simulink model "Filter_testaus_uusi"  (R2017b)
settings: Solver=FixedStepDiscrete  StartTime=0.0  StopTime=10  FixedStep=1/44100  RelTol=1e-3
(part 3 of 4)

== system Filter_testaus_uusi/Highpass/HighpassH/Resonator30 ==
  In1 : Inport
  Constant : Constant  Value=0i
  Delay : Delay  DelayLength=1
  Gain : Gain  Gain=0.0139+0.9999i
  GainH : Gain  Gain=-0.7217-0.69221i
  Real-Imag to Complex : RealImagToComplex
  Sum1 : Sum  Inputs=|++
  Out1 : Outport
  wires:
  Constant/1 -> Real-Imag to Complex/2
  Real-Imag to Complex/1 -> Sum1/1
  In1/1 -> Real-Imag to Complex/1
  GainH/1 -> Out1/1
  Gain/1 -> Sum1/2
  Delay/1 -> Gain/1
  Sum1/1 -> Delay/1, GainH/1

== system Filter_testaus_uusi/Highpass/HighpassH/Resonator31 ==
  In1 : Inport
  Constant : Constant  Value=0i
  Delay : Delay  DelayLength=1
  Gain : Gain  Gain=-0.0139+0.9999i
  GainH : Gain  Gain=0.712+0.70218i
  Real-Imag to Complex : RealImagToComplex
  Sum1 : Sum  Inputs=|++
  Out1 : Outport
  wires:
  Constant/1 -> Real-Imag to Complex/2
  Real-Imag to Complex/1 -> Sum1/1
  In1/1 -> Real-Imag to Complex/1
  GainH/1 -> Out1/1
  Gain/1 -> Sum1/2
  Delay/1 -> Gain/1
  Sum1/1 -> Delay/1, GainH/1

== system Filter_testaus_uusi/Highpass/HighpassH/Resonator32 ==
  In1 : Inport
  Constant : Constant  Value=0i
  Delay : Delay  DelayLength=1
  Gain : Gain  Gain=-0.04169+0.99913i
  GainH : Gain  Gain=-0.70218-0.712i
  Real-Imag to Complex : RealImagToComplex
  Sum1 : Sum  Inputs=|++
  Out1 : Outport
  wires:
  Constant/1 -> Real-Imag to Complex/2
  Real-Imag to Complex/1 -> Sum1/1
  In1/1 -> Real-Imag to Complex/1
  GainH/1 -> Out1/1
  Gain/1 -> Sum1/2
  Delay/1 -> Gain/1
  Sum1/1 -> Delay/1, GainH/1

== system Filter_testaus_uusi/Highpass/HighpassH/Resonator33 ==
  In1 : Inport
  Constant : Constant  Value=0i
  Delay : Delay  DelayLength=1
  Gain : Gain  Gain=-0.069448+0.99759i
  GainH : Gain  Gain=0.69221+0.7217i
  Real-Imag to Complex : RealImagToComplex
  Sum1 : Sum  Inputs=|++
  Out1 : Outport
  wires:
  Constant/1 -> Real-Imag to Complex/2
  Real-Imag to Complex/1 -> Sum1/1
  In1/1 -> Real-Imag to Complex/1
  GainH/1 -> Out1/1
  Gain/1 -> Sum1/2
  Delay/1 -> Gain/1
  Sum1/1 -> Delay/1, GainH/1

== system Filter_testaus_uusi/Highpass/HighpassH/Resonator34 ==
  In1 : Inport
  Constant : Constant  Value=0i
  Delay : Delay  DelayLength=1
  Gain : Gain  Gain=-0.097152+0.99527i
  GainH : Gain  Gain=-0.68211-0.73125i
  Real-Imag to Complex : RealImagToComplex
  Sum1 : Sum  Inputs=|++
  Out1 : Outport
  wires:
  Constant/1 -> Real-Imag to Complex/2
  Real-Imag to Complex/1 -> Sum1/1
  In1/1 -> Real-Imag to Complex/1
  GainH/1 -> Out1/1
  Gain/1 -> Sum1/2
  Delay/1 -> Gain/1
  Sum1/1 -> Delay/1, GainH/1

== system Filter_testaus_uusi/Highpass/HighpassH/Resonator35 ==
  In1 : Inport
  Constant : Constant  Value=0i
  Delay : Delay  DelayLength=1
  Gain : Gain  Gain=-0.12478+0.99218i
  GainH : Gain  Gain=0.67188+0.74066i
  Real-Imag to Complex : RealImagToComplex
  Sum1 : Sum  Inputs=|++
  Out1 : Outport
  wires:
  Constant/1 -> Real-Imag to Complex/2
  Real-Imag to Complex/1 -> Sum1/1
  In1/1 -> Real-Imag to Complex/1
  GainH/1 -> Out1/1
  Gain/1 -> Sum1/2
  Delay/1 -> Gain/1
  Sum1/1 -> Delay/1, GainH/1

== system Filter_testaus_uusi/Highpass/HighpassH/Resonator36 ==
  In1 : Inport
  Constant : Constant  Value=0i
  Delay : Delay  DelayLength=1
  Gain : Gain  Gain=-0.15231+0.98833i
  GainH : Gain  Gain=-0.66152-0.74993i
  Real-Imag to Complex : RealImagToComplex
  Sum1 : Sum  Inputs=|++
  Out1 : Outport
  wires:
  Constant/1 -> Real-Imag to Complex/2
  Real-Imag to Complex/1 -> Sum1/1
  In1/1 -> Real-Imag to Complex/1
  GainH/1 -> Out1/1
  Gain/1 -> Sum1/2
  Delay/1 -> Gain/1
  Sum1/1 -> Delay/1, GainH/1

== system Filter_testaus_uusi/Highpass/HighpassH/Resonator37 ==
  In1 : Inport
  Constant : Constant  Value=0i
  Delay : Delay  DelayLength=1
  Gain : Gain  Gain=-0.17973+0.98372i
  GainH : Gain  Gain=0.65103+0.75905i
  Real-Imag to Complex : RealImagToComplex
  Sum1 : Sum  Inputs=|++
  Out1 : Outport
  wires:
  Constant/1 -> Real-Imag to Complex/2
  Real-Imag to Complex/1 -> Sum1/1
  In1/1 -> Real-Imag to Complex/1
  GainH/1 -> Out1/1
  Gain/1 -> Sum1/2
  Delay/1 -> Gain/1
  Sum1/1 -> Delay/1, GainH/1

== system Filter_testaus_uusi/Highpass/HighpassH/Resonator38 ==
  In1 : Inport
  Constant : Constant  Value=0i
  Delay : Delay  DelayLength=1
  Gain : Gain  Gain=-0.20701+0.97834i
  GainH : Gain  Gain=-0.64042-0.76803i
  Real-Imag to Complex : RealImagToComplex
  Sum1 : Sum  Inputs=|++
  Out1 : Outport
  wires:
  Constant/1 -> Real-Imag to Complex/2
  Real-Imag to Complex/1 -> Sum1/1
  In1/1 -> Real-Imag to Complex/1
  GainH/1 -> Out1/1
  Gain/1 -> Sum1/2
  Delay/1 -> Gain/1
  Sum1/1 -> Delay/1, GainH/1

== system Filter_testaus_uusi/Highpass/HighpassH/Resonator39 ==
  In1 : Inport
  Constant : Constant  Value=0i
  Delay : Delay  DelayLength=1
  Gain : Gain  Gain=-0.23412+0.97221i
  GainH : Gain  Gain=0.62968+0.77685i
  Real-Imag to Complex : RealImagToComplex
  Sum1 : Sum  Inputs=|++
  Out1 : Outport
  wires:
  Constant/1 -> Real-Imag to Complex/2
  Real-Imag to Complex/1 -> Sum1/1
  In1/1 -> Real-Imag to Complex/1
  GainH/1 -> Out1/1
  Gain/1 -> Sum1/2
  Delay/1 -> Gain/1
  Sum1/1 -> Delay/1, GainH/1

== system Filter_testaus_uusi/Highpass/HighpassH/Resonator4 ==
  In1 : Inport
  Constant : Constant  Value=0i
  Delay : Delay  DelayLength=1
  Gain : Gain  Gain=0.67188+0.74066i
  GainH : Gain  Gain=-0.91984-0.39229i
  Real-Imag to Complex : RealImagToComplex
  Sum1 : Sum  Inputs=|++
  Out1 : Outport
  wires:
  Constant/1 -> Real-Imag to Complex/2
  Real-Imag to Complex/1 -> Sum1/1
  In1/1 -> Real-Imag to Complex/1
  GainH/1 -> Out1/1
  Gain/1 -> Sum1/2
  Delay/1 -> Gain/1
  Sum1/1 -> Delay/1, GainH/1

== system Filter_testaus_uusi/Highpass/HighpassH/Resonator40 ==
  In1 : Inport
  Constant : Constant  Value=0i
  Delay : Delay  DelayLength=1
  Gain : Gain  Gain=-0.26106+0.96532i
  GainH : Gain  Gain=-0.61882-0.78553i
  Real-Imag to Complex : RealImagToComplex
  Sum1 : Sum  Inputs=|++
  Out1 : Outport
  wires:
  Constant/1 -> Real-Imag to Complex/2
  Real-Imag to Complex/1 -> Sum1/1
  In1/1 -> Real-Imag to Complex/1
  GainH/1 -> Out1/1
  Gain/1 -> Sum1/2
  Delay/1 -> Gain/1
  Sum1/1 -> Delay/1, GainH/1

== system Filter_testaus_uusi/Highpass/HighpassH/Resonator41 ==
  In1 : Inport
  Constant : Constant  Value=0i
  Delay : Delay  DelayLength=1
  Gain : Gain  Gain=-0.28779+0.95769i
  GainH : Gain  Gain=0.60784+0.79406i
  Real-Imag to Complex : RealImagToComplex
  Sum1 : Sum  Inputs=|++
  Out1 : Outport
  wires:
  Constant/1 -> Real-Imag to Complex/2
  Real-Imag to Complex/1 -> Sum1/1
  In1/1 -> Real-Imag to Complex/1
  GainH/1 -> Out1/1
  Gain/1 -> Sum1/2
  Delay/1 -> Gain/1
  Sum1/1 -> Delay/1, GainH/1

== system Filter_testaus_uusi/Highpass/HighpassH/Resonator42 ==
  In1 : Inport
  Constant : Constant  Value=0i
  Delay : Delay  DelayLength=1
  Gain : Gain  Gain=-0.3143+0.94932i
  GainH : Gain  Gain=-0.59675-0.80243i
  Real-Imag to Complex : RealImagToComplex
  Sum1 : Sum  Inputs=|++
  Out1 : Outport
  wires:
  Constant/1 -> Real-Imag to Complex/2
  Real-Imag to Complex/1 -> Sum1/1
  In1/1 -> Real-Imag to Complex/1
  GainH/1 -> Out1/1
  Gain/1 -> Sum1/2
  Delay/1 -> Gain/1
  Sum1/1 -> Delay/1, GainH/1

== system Filter_testaus_uusi/Highpass/HighpassH/Resonator43 ==
  In1 : Inport
  Constant : Constant  Value=0i
  Delay : Delay  DelayLength=1
  Gain : Gain  Gain=-0.34057+0.94022i
  GainH : Gain  Gain=0.58553+0.81065i
  Real-Imag to Complex : RealImagToComplex
  Sum1 : Sum  Inputs=|++
  Out1 : Outport
  wires:
  Constant/1 -> Real-Imag to Complex/2
  Real-Imag to Complex/1 -> Sum1/1
  In1/1 -> Real-Imag to Complex/1
  GainH/1 -> Out1/1
  Gain/1 -> Sum1/2
  Delay/1 -> Gain/1
  Sum1/1 -> Delay/1, GainH/1

== system Filter_testaus_uusi/Highpass/HighpassH/Resonator44 ==
  In1 : Inport
  Constant : Constant  Value=0i
  Delay : Delay  DelayLength=1
  Gain : Gain  Gain=-0.36657+0.93039i
  GainH : Gain  Gain=-0.57421-0.81871i
  Real-Imag to Complex : RealImagToComplex
  Sum1 : Sum  Inputs=|++
  Out1 : Outport
  wires:
  Constant/1 -> Real-Imag to Complex/2
  Real-Imag to Complex/1 -> Sum1/1
  In1/1 -> Real-Imag to Complex/1
  GainH/1 -> Out1/1
  Gain/1 -> Sum1/2
  Delay/1 -> Gain/1
  Sum1/1 -> Delay/1, GainH/1

== system Filter_testaus_uusi/Highpass/HighpassH/Resonator45 ==
  In1 : Inport
  Constant : Constant  Value=0i
  Delay : Delay  DelayLength=1
  Gain : Gain  Gain=-0.39229+0.91984i
  GainH : Gain  Gain=0.56277+0.82661i
  Real-Imag to Complex : RealImagToComplex
  Sum1 : Sum  Inputs=|++
  Out1 : Outport
  wires:
  Constant/1 -> Real-Imag to Complex/2
  Real-Imag to Complex/1 -> Sum1/1
  In1/1 -> Real-Imag to Complex/1
  GainH/1 -> Out1/1
  Gain/1 -> Sum1/2
  Delay/1 -> Gain/1
  Sum1/1 -> Delay/1, GainH/1

== system Filter_testaus_uusi/Highpass/HighpassH/Resonator46 ==
  In1 : Inport
  Constant : Constant  Value=0i
  Delay : Delay  DelayLength=1
  Gain : Gain  Gain=-0.41771+0.90858i
  GainH : Gain  Gain=-0.55123-0.83435i
  Real-Imag to Complex : RealImagToComplex
  Sum1 : Sum  Inputs=|++
  Out1 : Outport
  wires:
  Constant/1 -> Real-Imag to Complex/2
  Real-Imag to Complex/1 -> Sum1/1
  In1/1 -> Real-Imag to Complex/1
  GainH/1 -> Out1/1
  Gain/1 -> Sum1/2
  Delay/1 -> Gain/1
  Sum1/1 -> Delay/1, GainH/1

== system Filter_testaus_uusi/Highpass/HighpassH/Resonator47 ==
  In1 : Inport
  Constant : Constant  Value=0i
  Delay : Delay  DelayLength=1
  Gain : Gain  Gain=-0.44281+0.89662i
  GainH : Gain  Gain=0.53958+0.84194i
  Real-Imag to Complex : RealImagToComplex
  Sum1 : Sum  Inputs=|++
  Out1 : Outport
  wires:
  Constant/1 -> Real-Imag to Complex/2
  Real-Imag to Complex/1 -> Sum1/1
  In1/1 -> Real-Imag to Complex/1
  GainH/1 -> Out1/1
  Gain/1 -> Sum1/2
  Delay/1 -> Gain/1
  Sum1/1 -> Delay/1, GainH/1

== system Filter_testaus_uusi/Highpass/HighpassH/Resonator48 ==
  In1 : Inport
  Constant : Constant  Value=0i
  Delay : Delay  DelayLength=1
  Gain : Gain  Gain=-0.46756+0.88396i
  GainH : Gain  Gain=-0.52782-0.84936i
  Real-Imag to Complex : RealImagToComplex
  Sum1 : Sum  Inputs=|++
  Out1 : Outport
  wires:
  Constant/1 -> Real-Imag to Complex/2
  Real-Imag to Complex/1 -> Sum1/1
  In1/1 -> Real-Imag to Complex/1
  GainH/1 -> Out1/1
  Gain/1 -> Sum1/2
  Delay/1 -> Gain/1
  Sum1/1 -> Delay/1, GainH/1

== system Filter_testaus_uusi/Highpass/HighpassH/Resonator49 ==
  In1 : Inport
  Constant : Constant  Value=0i
  Delay : Delay  DelayLength=1
  Gain : Gain  Gain=-0.49195+0.87062i
  GainH : Gain  Gain=0.51596+0.85661i
  Real-Imag to Complex : RealImagToComplex
  Sum1 : Sum  Inputs=|++
  Out1 : Outport
  wires:
  Constant/1 -> Real-Imag to Complex/2
  Real-Imag to Complex/1 -> Sum1/1
  In1/1 -> Real-Imag to Complex/1
  GainH/1 -> Out1/1
  Gain/1 -> Sum1/2
  Delay/1 -> Gain/1
  Sum1/1 -> Delay/1, GainH/1

== system Filter_testaus_uusi/Highpass/HighpassH/Resonator5 ==
  In1 : Inport
  Constant : Constant  Value=0i
  Delay : Delay  DelayLength=1
  Gain : Gain  Gain=0.65103+0.75905i
  GainH : Gain  Gain=0.9143+0.40504i
  Real-Imag to Complex : RealImagToComplex
  Sum1 : Sum  Inputs=|++
  Out1 : Outport
  wires:
  Constant/1 -> Real-Imag to Complex/2
  Real-Imag to Complex/1 -> Sum1/1
  In1/1 -> Real-Imag to Complex/1
  GainH/1 -> Out1/1
  Gain/1 -> Sum1/2
  Delay/1 -> Gain/1
  Sum1/1 -> Delay/1, GainH/1

== system Filter_testaus_uusi/Highpass/HighpassH/Resonator50 ==
  In1 : Inport
  Constant : Constant  Value=0i
  Delay : Delay  DelayLength=1
  Gain : Gain  Gain=-0.51596+0.85661i
  GainH : Gain  Gain=-0.50401-0.8637i
  Real-Imag to Complex : RealImagToComplex
  Sum1 : Sum  Inputs=|++
  Out1 : Outport
  wires:
  Constant/1 -> Real-Imag to Complex/2
  Real-Imag to Complex/1 -> Sum1/1
  In1/1 -> Real-Imag to Complex/1
  GainH/1 -> Out1/1
  Gain/1 -> Sum1/2
  Delay/1 -> Gain/1
  Sum1/1 -> Delay/1, GainH/1

== system Filter_testaus_uusi/Highpass/HighpassH/Resonator51 ==
  In1 : Inport
  Constant : Constant  Value=0i
  Delay : Delay  DelayLength=1
  Gain : Gain  Gain=-0.53958+0.84194i
  GainH : Gain  Gain=0.49195+0.87062i
  Real-Imag to Complex : RealImagToComplex
  Sum1 : Sum  Inputs=|++
  Out1 : Outport
  wires:
  Constant/1 -> Real-Imag to Complex/2
  Real-Imag to Complex/1 -> Sum1/1
  In1/1 -> Real-Imag to Complex/1
  GainH/1 -> Out1/1
  Gain/1 -> Sum1/2
  Delay/1 -> Gain/1
  Sum1/1 -> Delay/1, GainH/1

== system Filter_testaus_uusi/Highpass/HighpassH/Resonator52 ==
  In1 : Inport
  Constant : Constant  Value=0i
  Delay : Delay  DelayLength=1
  Gain : Gain  Gain=-0.56277+0.82661i
  GainH : Gain  Gain=-0.4798-0.87738i
  Real-Imag to Complex : RealImagToComplex
  Sum1 : Sum  Inputs=|++
  Out1 : Outport
  wires:
  Constant/1 -> Real-Imag to Complex/2
  Real-Imag to Complex/1 -> Sum1/1
  In1/1 -> Real-Imag to Complex/1
  GainH/1 -> Out1/1
  Gain/1 -> Sum1/2
  Delay/1 -> Gain/1
  Sum1/1 -> Delay/1, GainH/1

== system Filter_testaus_uusi/Highpass/HighpassH/Resonator53 ==
  In1 : Inport
  Constant : Constant  Value=0i
  Delay : Delay  DelayLength=1
  Gain : Gain  Gain=-0.58553+0.81065i
  GainH : Gain  Gain=0.46756+0.88396i
  Real-Imag to Complex : RealImagToComplex
  Sum1 : Sum  Inputs=|++
  Out1 : Outport
  wires:
  Constant/1 -> Real-Imag to Complex/2
  Real-Imag to Complex/1 -> Sum1/1
  In1/1 -> Real-Imag to Complex/1
  GainH/1 -> Out1/1
  Gain/1 -> Sum1/2
  Delay/1 -> Gain/1
  Sum1/1 -> Delay/1, GainH/1

== system Filter_testaus_uusi/Highpass/HighpassH/Resonator54 ==
  In1 : Inport
  Constant : Constant  Value=0i
  Delay : Delay  DelayLength=1
  Gain : Gain  Gain=-0.60784+0.79406i
  GainH : Gain  Gain=-0.45523-0.89037i
  Real-Imag to Complex : RealImagToComplex
  Sum1 : Sum  Inputs=|++
  Out1 : Outport
  wires:
  Constant/1 -> Real-Imag to Complex/2
  Real-Imag to Complex/1 -> Sum1/1
  In1/1 -> Real-Imag to Complex/1
  GainH/1 -> Out1/1
  Gain/1 -> Sum1/2
  Delay/1 -> Gain/1
  Sum1/1 -> Delay/1, GainH/1

== system Filter_testaus_uusi/Highpass/HighpassH/Resonator55 ==
  In1 : Inport
  Constant : Constant  Value=0i
  Delay : Delay  DelayLength=1
  Gain : Gain  Gain=-0.62968+0.77685i
  GainH : Gain  Gain=0.44281+0.89662i
  Real-Imag to Complex : RealImagToComplex
  Sum1 : Sum  Inputs=|++
  Out1 : Outport
  wires:
  Constant/1 -> Real-Imag to Complex/2
  Real-Imag to Complex/1 -> Sum1/1
  In1/1 -> Real-Imag to Complex/1
  GainH/1 -> Out1/1
  Gain/1 -> Sum1/2
  Delay/1 -> Gain/1
  Sum1/1 -> Delay/1, GainH/1

== system Filter_testaus_uusi/Highpass/HighpassH/Resonator56 ==
  In1 : Inport
  Constant : Constant  Value=0i
  Delay : Delay  DelayLength=1
  Gain : Gain  Gain=-0.65103+0.75905i
  GainH : Gain  Gain=-0.4303-0.90269i
  Real-Imag to Complex : RealImagToComplex
  Sum1 : Sum  Inputs=|++
  Out1 : Outport
  wires:
  Constant/1 -> Real-Imag to Complex/2
  Real-Imag to Complex/1 -> Sum1/1
  In1/1 -> Real-Imag to Complex/1
  GainH/1 -> Out1/1
  Gain/1 -> Sum1/2
  Delay/1 -> Gain/1
  Sum1/1 -> Delay/1, GainH/1

== system Filter_testaus_uusi/Highpass/HighpassH/Resonator57 ==
  In1 : Inport
  Constant : Constant  Value=0i
  Delay : Delay  DelayLength=1
  Gain : Gain  Gain=-0.67188+0.74066i
  GainH : Gain  Gain=0.41771+0.90858i
  Real-Imag to Complex : RealImagToComplex
  Sum1 : Sum  Inputs=|++
  Out1 : Outport
  wires:
  Constant/1 -> Real-Imag to Complex/2
  Real-Imag to Complex/1 -> Sum1/1
  In1/1 -> Real-Imag to Complex/1
  GainH/1 -> Out1/1
  Gain/1 -> Sum1/2
  Delay/1 -> Gain/1
  Sum1/1 -> Delay/1, GainH/1

== system Filter_testaus_uusi/Highpass/HighpassH/Resonator58 ==
  In1 : Inport
  Constant : Constant  Value=0i
  Delay : Delay  DelayLength=1
  Gain : Gain  Gain=-0.69221+0.7217i
  GainH : Gain  Gain=-0.40504-0.9143i
  Real-Imag to Complex : RealImagToComplex
  Sum1 : Sum  Inputs=|++
  Out1 : Outport
  wires:
  Constant/1 -> Real-Imag to Complex/2
  Real-Imag to Complex/1 -> Sum1/1
  In1/1 -> Real-Imag to Complex/1
  GainH/1 -> Out1/1
  Gain/1 -> Sum1/2
  Delay/1 -> Gain/1
  Sum1/1 -> Delay/1, GainH/1

== system Filter_testaus_uusi/Highpass/HighpassH/Resonator59 ==
  In1 : Inport
  Constant : Constant  Value=0i
  Delay : Delay  DelayLength=1
  Gain : Gain  Gain=-0.712+0.70218i
  GainH : Gain  Gain=0.39229+0.91984i
  Real-Imag to Complex : RealImagToComplex
  Sum1 : Sum  Inputs=|++
  Out1 : Outport
  wires:
  Constant/1 -> Real-Imag to Complex/2
  Real-Imag to Complex/1 -> Sum1/1
  In1/1 -> Real-Imag to Complex/1
  GainH/1 -> Out1/1
  Gain/1 -> Sum1/2
  Delay/1 -> Gain/1
  Sum1/1 -> Delay/1, GainH/1

== system Filter_testaus_uusi/Highpass/HighpassH/Resonator6 ==
  In1 : Inport
  Constant : Constant  Value=0i
  Delay : Delay  DelayLength=1
  Gain : Gain  Gain=0.62968+0.77685i
  GainH : Gain  Gain=-0.90858-0.41771i
  Real-Imag to Complex : RealImagToComplex
  Sum1 : Sum  Inputs=|++
  Out1 : Outport
  wires:
  Constant/1 -> Real-Imag to Complex/2
  Real-Imag to Complex/1 -> Sum1/1
  In1/1 -> Real-Imag to Complex/1
  GainH/1 -> Out1/1
  Gain/1 -> Sum1/2
  Delay/1 -> Gain/1
  Sum1/1 -> Delay/1, GainH/1

== system Filter_testaus_uusi/Highpass/HighpassH/Resonator60 ==
  In1 : Inport
  Constant : Constant  Value=0i
  Delay : Delay  DelayLength=1
  Gain : Gain  Gain=-0.73125+0.68211i
  GainH : Gain  Gain=-0.37947-0.9252i
  Real-Imag to Complex : RealImagToComplex
  Sum1 : Sum  Inputs=|++
  Out1 : Outport
  wires:
  Constant/1 -> Real-Imag to Complex/2
  Real-Imag to Complex/1 -> Sum1/1
  In1/1 -> Real-Imag to Complex/1
  GainH/1 -> Out1/1
  Gain/1 -> Sum1/2
  Delay/1 -> Gain/1
  Sum1/1 -> Delay/1, GainH/1

== system Filter_testaus_uusi/Highpass/HighpassH/Resonator61 ==
  In1 : Inport
  Constant : Constant  Value=0i
  Delay : Delay  DelayLength=1
  Gain : Gain  Gain=-0.74993+0.66152i
  GainH : Gain  Gain=0.36657+0.93039i
  Real-Imag to Complex : RealImagToComplex
  Sum1 : Sum  Inputs=|++
  Out1 : Outport
  wires:
  Constant/1 -> Real-Imag to Complex/2
  Real-Imag to Complex/1 -> Sum1/1
  In1/1 -> Real-Imag to Complex/1
  GainH/1 -> Out1/1
  Gain/1 -> Sum1/2
  Delay/1 -> Gain/1
  Sum1/1 -> Delay/1, GainH/1

== system Filter_testaus_uusi/Highpass/HighpassH/Resonator62 ==
  In1 : Inport
  Constant : Constant  Value=0i
  Delay : Delay  DelayLength=1
  Gain : Gain  Gain=-0.76803+0.64042i
  GainH : Gain  Gain=-0.3536-0.93539i
  Real-Imag to Complex : RealImagToComplex
  Sum1 : Sum  Inputs=|++
  Out1 : Outport
  wires:
  Constant/1 -> Real-Imag to Complex/2
  Real-Imag to Complex/1 -> Sum1/1
  In1/1 -> Real-Imag to Complex/1
  GainH/1 -> Out1/1
  Gain/1 -> Sum1/2
  Delay/1 -> Gain/1
  Sum1/1 -> Delay/1, GainH/1

== system Filter_testaus_uusi/Highpass/HighpassH/Resonator63 ==
  In1 : Inport
  Constant : Constant  Value=0i
  Delay : Delay  DelayLength=1
  Gain : Gain  Gain=-0.78553+0.61882i
  GainH : Gain  Gain=0.34057+0.94022i
  Real-Imag to Complex : RealImagToComplex
  Sum1 : Sum  Inputs=|++
  Out1 : Outport
  wires:
  Constant/1 -> Real-Imag to Complex/2
  Real-Imag to Complex/1 -> Sum1/1
  In1/1 -> Real-Imag to Complex/1
  GainH/1 -> Out1/1
  Gain/1 -> Sum1/2
  Delay/1 -> Gain/1
  Sum1/1 -> Delay/1, GainH/1

== system Filter_testaus_uusi/Highpass/HighpassH/Resonator64 ==
  In1 : Inport
  Constant : Constant  Value=0i
  Delay : Delay  DelayLength=1
  Gain : Gain  Gain=-0.80243+0.59675i
  GainH : Gain  Gain=-0.32747-0.94486i
  Real-Imag to Complex : RealImagToComplex
  Sum1 : Sum  Inputs=|++
  Out1 : Outport
  wires:
  Constant/1 -> Real-Imag to Complex/2
  Real-Imag to Complex/1 -> Sum1/1
  In1/1 -> Real-Imag to Complex/1
  GainH/1 -> Out1/1
  Gain/1 -> Sum1/2
  Delay/1 -> Gain/1
  Sum1/1 -> Delay/1, GainH/1

== system Filter_testaus_uusi/Highpass/HighpassH/Resonator65 ==
  In1 : Inport
  Constant : Constant  Value=0i
  Delay : Delay  DelayLength=1
  Gain : Gain  Gain=-0.81871+0.57421i
  GainH : Gain  Gain=0.3143+0.94932i
  Real-Imag to Complex : RealImagToComplex
  Sum1 : Sum  Inputs=|++
  Out1 : Outport
  wires:
  Constant/1 -> Real-Imag to Complex/2
  Real-Imag to Complex/1 -> Sum1/1
  In1/1 -> Real-Imag to Complex/1
  GainH/1 -> Out1/1
  Gain/1 -> Sum1/2
  Delay/1 -> Gain/1
  Sum1/1 -> Delay/1, GainH/1

== system Filter_testaus_uusi/Highpass/HighpassH/Resonator66 ==
  In1 : Inport
  Constant : Constant  Value=0i
  Delay : Delay  DelayLength=1
  Gain : Gain  Gain=-0.83435+0.55123i
  GainH : Gain  Gain=-0.30107-0.9536i
  Real-Imag to Complex : RealImagToComplex
  Sum1 : Sum  Inputs=|++
  Out1 : Outport
  wires:
  Constant/1 -> Real-Imag to Complex/2
  Real-Imag to Complex/1 -> Sum1/1
  In1/1 -> Real-Imag to Complex/1
  GainH/1 -> Out1/1
  Gain/1 -> Sum1/2
  Delay/1 -> Gain/1
  Sum1/1 -> Delay/1, GainH/1

== system Filter_testaus_uusi/Highpass/HighpassH/Resonator67 ==
  In1 : Inport
  Constant : Constant  Value=0i
  Delay : Delay  DelayLength=1
  Gain : Gain  Gain=-0.84936+0.52782i
  GainH : Gain  Gain=0.28779+0.95769i
  Real-Imag to Complex : RealImagToComplex
  Sum1 : Sum  Inputs=|++
  Out1 : Outport
  wires:
  Constant/1 -> Real-Imag to Complex/2
  Real-Imag to Complex/1 -> Sum1/1
  In1/1 -> Real-Imag to Complex/1
  GainH/1 -> Out1/1
  Gain/1 -> Sum1/2
  Delay/1 -> Gain/1
  Sum1/1 -> Delay/1, GainH/1

== system Filter_testaus_uusi/Highpass/HighpassH/Resonator68 ==
  In1 : Inport
  Constant : Constant  Value=0i
  Delay : Delay  DelayLength=1
  Gain : Gain  Gain=-0.8637+0.50401i
  GainH : Gain  Gain=-0.27445-0.9616i
  Real-Imag to Complex : RealImagToComplex
  Sum1 : Sum  Inputs=|++
  Out1 : Outport
  wires:
  Constant/1 -> Real-Imag to Complex/2
  Real-Imag to Complex/1 -> Sum1/1
  In1/1 -> Real-Imag to Complex/1
  GainH/1 -> Out1/1
  Gain/1 -> Sum1/2
  Delay/1 -> Gain/1
  Sum1/1 -> Delay/1, GainH/1

== system Filter_testaus_uusi/Highpass/HighpassH/Resonator69 ==
  In1 : Inport
  Constant : Constant  Value=0i
  Delay : Delay  DelayLength=1
  Gain : Gain  Gain=-0.87738+0.4798i
  GainH : Gain  Gain=0.26106+0.96532i
  Real-Imag to Complex : RealImagToComplex
  Sum1 : Sum  Inputs=|++
  Out1 : Outport
  wires:
  Constant/1 -> Real-Imag to Complex/2
  Real-Imag to Complex/1 -> Sum1/1
  In1/1 -> Real-Imag to Complex/1
  GainH/1 -> Out1/1
  Gain/1 -> Sum1/2
  Delay/1 -> Gain/1
  Sum1/1 -> Delay/1, GainH/1

== system Filter_testaus_uusi/Highpass/HighpassH/Resonator7 ==
  In1 : Inport
  Constant : Constant  Value=0i
  Delay : Delay  DelayLength=1
  Gain : Gain  Gain=0.60784+0.79406i
  GainH : Gain  Gain=0.90269+0.4303i
  Real-Imag to Complex : RealImagToComplex
  Sum1 : Sum  Inputs=|++
  Out1 : Outport
  wires:
  Constant/1 -> Real-Imag to Complex/2
  Real-Imag to Complex/1 -> Sum1/1
  In1/1 -> Real-Imag to Complex/1
  GainH/1 -> Out1/1
  Gain/1 -> Sum1/2
  Delay/1 -> Gain/1
  Sum1/1 -> Delay/1, GainH/1

== system Filter_testaus_uusi/Highpass/HighpassH/Resonator70 ==
  In1 : Inport
  Constant : Constant  Value=0i
  Delay : Delay  DelayLength=1
  Gain : Gain  Gain=-0.89037+0.45523i
  GainH : Gain  Gain=-0.24761-0.96886i
  Real-Imag to Complex : RealImagToComplex
  Sum1 : Sum  Inputs=|++
  Out1 : Outport
  wires:
  Constant/1 -> Real-Imag to Complex/2
  Real-Imag to Complex/1 -> Sum1/1
  In1/1 -> Real-Imag to Complex/1
  GainH/1 -> Out1/1
  Gain/1 -> Sum1/2
  Delay/1 -> Gain/1
  Sum1/1 -> Delay/1, GainH/1

== system Filter_testaus_uusi/Highpass/HighpassH/Resonator71 ==
  In1 : Inport
  Constant : Constant  Value=0i
  Delay : Delay  DelayLength=1
  Gain : Gain  Gain=-0.90269+0.4303i
  GainH : Gain  Gain=0.23412+0.97221i
  Real-Imag to Complex : RealImagToComplex
  Sum1 : Sum  Inputs=|++
  Out1 : Outport
  wires:
  Constant/1 -> Real-Imag to Complex/2
  Real-Imag to Complex/1 -> Sum1/1
  In1/1 -> Real-Imag to Complex/1
  GainH/1 -> Out1/1
  Gain/1 -> Sum1/2
  Delay/1 -> Gain/1
  Sum1/1 -> Delay/1, GainH/1

== system Filter_testaus_uusi/Highpass/HighpassH/Resonator72 ==
  In1 : Inport
  Constant : Constant  Value=0i
  Delay : Delay  DelayLength=1
  Gain : Gain  Gain=-0.9143+0.40504i
  GainH : Gain  Gain=-0.22058-0.97537i
  Real-Imag to Complex : RealImagToComplex
  Sum1 : Sum  Inputs=|++
  Out1 : Outport
  wires:
  Constant/1 -> Real-Imag to Complex/2
  Real-Imag to Complex/1 -> Sum1/1
  In1/1 -> Real-Imag to Complex/1
  GainH/1 -> Out1/1
  Gain/1 -> Sum1/2
  Delay/1 -> Gain/1
  Sum1/1 -> Delay/1, GainH/1

== system Filter_testaus_uusi/Highpass/HighpassH/Resonator73 ==
  In1 : Inport
  Constant : Constant  Value=0i
  Delay : Delay  DelayLength=1
  Gain : Gain  Gain=-0.9252+0.37947i
  GainH : Gain  Gain=0.20701+0.97834i
  Real-Imag to Complex : RealImagToComplex
  Sum1 : Sum  Inputs=|++
  Out1 : Outport
  wires:
  Constant/1 -> Real-Imag to Complex/2
  Real-Imag to Complex/1 -> Sum1/1
  In1/1 -> Real-Imag to Complex/1
  GainH/1 -> Out1/1
  Gain/1 -> Sum1/2
  Delay/1 -> Gain/1
  Sum1/1 -> Delay/1, GainH/1

== system Filter_testaus_uusi/Highpass/HighpassH/Resonator74 ==
  In1 : Inport
  Constant : Constant  Value=0i
  Delay : Delay  DelayLength=1
  Gain : Gain  Gain=-0.93539+0.3536i
  GainH : Gain  Gain=-0.19339-0.98112i
  Real-Imag to Complex : RealImagToComplex
  Sum1 : Sum  Inputs=|++
  Out1 : Outport
  wires:
  Constant/1 -> Real-Imag to Complex/2
  Real-Imag to Complex/1 -> Sum1/1
  In1/1 -> Real-Imag to Complex/1
  GainH/1 -> Out1/1
  Gain/1 -> Sum1/2
  Delay/1 -> Gain/1
  Sum1/1 -> Delay/1, GainH/1

== system Filter_testaus_uusi/Highpass/HighpassH/Resonator75 ==
  In1 : Inport
  Constant : Constant  Value=0i
  Delay : Delay  DelayLength=1
  Gain : Gain  Gain=-0.94486+0.32747i
  GainH : Gain  Gain=0.17973+0.98372i
  Real-Imag to Complex : RealImagToComplex
  Sum1 : Sum  Inputs=|++
  Out1 : Outport
  wires:
  Constant/1 -> Real-Imag to Complex/2
  Real-Imag to Complex/1 -> Sum1/1
  In1/1 -> Real-Imag to Complex/1
  GainH/1 -> Out1/1
  Gain/1 -> Sum1/2
  Delay/1 -> Gain/1
  Sum1/1 -> Delay/1, GainH/1

== system Filter_testaus_uusi/Highpass/HighpassH/Resonator76 ==
  In1 : Inport
  Constant : Constant  Value=0i
  Delay : Delay  DelayLength=1
  Gain : Gain  Gain=-0.9536+0.30107i
  GainH : Gain  Gain=-0.16604-0.98612i
  Real-Imag to Complex : RealImagToComplex
  Sum1 : Sum  Inputs=|++
  Out1 : Outport
  wires:
  Constant/1 -> Real-Imag to Complex/2
  Real-Imag to Complex/1 -> Sum1/1
  In1/1 -> Real-Imag to Complex/1
  GainH/1 -> Out1/1
  Gain/1 -> Sum1/2
  Delay/1 -> Gain/1
  Sum1/1 -> Delay/1, GainH/1

== system Filter_testaus_uusi/Highpass/HighpassH/Resonator77 ==
  In1 : Inport
  Constant : Constant  Value=0i
  Delay : Delay  DelayLength=1
  Gain : Gain  Gain=-0.9616+0.27445i
  GainH : Gain  Gain=0.15231+0.98833i
  Real-Imag to Complex : RealImagToComplex
  Sum1 : Sum  Inputs=|++
  Out1 : Outport
  wires:
  Constant/1 -> Real-Imag to Complex/2
  Real-Imag to Complex/1 -> Sum1/1
  In1/1 -> Real-Imag to Complex/1
  GainH/1 -> Out1/1
  Gain/1 -> Sum1/2
  Delay/1 -> Gain/1
  Sum1/1 -> Delay/1, GainH/1

== system Filter_testaus_uusi/Highpass/HighpassH/Resonator78 ==
  In1 : Inport
  Constant : Constant  Value=0i
  Delay : Delay  DelayLength=1
  Gain : Gain  Gain=-0.96886+0.24761i
  GainH : Gain  Gain=-0.13856-0.99035i
  Real-Imag to Complex : RealImagToComplex
  Sum1 : Sum  Inputs=|++
  Out1 : Outport
  wires:
  Constant/1 -> Real-Imag to Complex/2
  Real-Imag to Complex/1 -> Sum1/1
  In1/1 -> Real-Imag to Complex/1
  GainH/1 -> Out1/1
  Gain/1 -> Sum1/2
  Delay/1 -> Gain/1
  Sum1/1 -> Delay/1, GainH/1

== system Filter_testaus_uusi/Highpass/HighpassH/Resonator79 ==
  In1 : Inport
  Constant : Constant  Value=0i
  Delay : Delay  DelayLength=1
  Gain : Gain  Gain=-0.97537+0.22058i
  GainH : Gain  Gain=0.12478+0.99218i
  Real-Imag to Complex : RealImagToComplex
  Sum1 : Sum  Inputs=|++
  Out1 : Outport
  wires:
  Constant/1 -> Real-Imag to Complex/2
  Real-Imag to Complex/1 -> Sum1/1
  In1/1 -> Real-Imag to Complex/1
  GainH/1 -> Out1/1
  Gain/1 -> Sum1/2
  Delay/1 -> Gain/1
  Sum1/1 -> Delay/1, GainH/1

== system Filter_testaus_uusi/Highpass/HighpassH/Resonator8 ==
  In1 : Inport
  Constant : Constant  Value=0i
  Delay : Delay  DelayLength=1
  Gain : Gain  Gain=0.58553+0.81065i
  GainH : Gain  Gain=-0.89662-0.44281i
  Real-Imag to Complex : RealImagToComplex
  Sum1 : Sum  Inputs=|++
  Out1 : Outport
  wires:
  Constant/1 -> Real-Imag to Complex/2
  Real-Imag to Complex/1 -> Sum1/1
  In1/1 -> Real-Imag to Complex/1
  GainH/1 -> Out1/1
  Gain/1 -> Sum1/2
  Delay/1 -> Gain/1
  Sum1/1 -> Delay/1, GainH/1

== system Filter_testaus_uusi/Highpass/HighpassH/Resonator80 ==
  In1 : Inport
  Constant : Constant  Value=0i
  Delay : Delay  DelayLength=1
  Gain : Gain  Gain=-0.98112+0.19339i
  GainH : Gain  Gain=-0.11098-0.99382i
  Real-Imag to Complex : RealImagToComplex
  Sum1 : Sum  Inputs=|++
  Out1 : Outport
  wires:
  Constant/1 -> Real-Imag to Complex/2
  Real-Imag to Complex/1 -> Sum1/1
  In1/1 -> Real-Imag to Complex/1
  GainH/1 -> Out1/1
  Gain/1 -> Sum1/2
  Delay/1 -> Gain/1
  Sum1/1 -> Delay/1, GainH/1

== system Filter_testaus_uusi/Highpass/HighpassH/Resonator81 ==
  In1 : Inport
  Constant : Constant  Value=0i
  Delay : Delay  DelayLength=1
  Gain : Gain  Gain=-0.98612+0.16604i
  GainH : Gain  Gain=0.097152+0.99527i
  Real-Imag to Complex : RealImagToComplex
  Sum1 : Sum  Inputs=|++
  Out1 : Outport
  wires:
  Constant/1 -> Real-Imag to Complex/2
  Real-Imag to Complex/1 -> Sum1/1
  In1/1 -> Real-Imag to Complex/1
  GainH/1 -> Out1/1
  Gain/1 -> Sum1/2
  Delay/1 -> Gain/1
  Sum1/1 -> Delay/1, GainH/1

== system Filter_testaus_uusi/Highpass/HighpassH/Resonator82 ==
  In1 : Inport
  Constant : Constant  Value=0i
  Delay : Delay  DelayLength=1
  Gain : Gain  Gain=-0.99035+0.13856i
  GainH : Gain  Gain=-0.083308-0.99652i
  Real-Imag to Complex : RealImagToComplex
  Sum1 : Sum  Inputs=|++
  Out1 : Outport
  wires:
  Constant/1 -> Real-Imag to Complex/2
  Real-Imag to Complex/1 -> Sum1/1
  In1/1 -> Real-Imag to Complex/1
  GainH/1 -> Out1/1
  Gain/1 -> Sum1/2
  Delay/1 -> Gain/1
  Sum1/1 -> Delay/1, GainH/1

== system Filter_testaus_uusi/Highpass/HighpassH/Resonator83 ==
  In1 : Inport
  Constant : Constant  Value=0i
  Delay : Delay  DelayLength=1
  Gain : Gain  Gain=-0.99382+0.11098i
  GainH : Gain  Gain=0.069448+0.99759i
  Real-Imag to Complex : RealImagToComplex
  Sum1 : Sum  Inputs=|++
  Out1 : Outport
  wires:
  Constant/1 -> Real-Imag to Complex/2
  Real-Imag to Complex/1 -> Sum1/1
  In1/1 -> Real-Imag to Complex/1
  GainH/1 -> Out1/1
  Gain/1 -> Sum1/2
  Delay/1 -> Gain/1
  Sum1/1 -> Delay/1, GainH/1

== system Filter_testaus_uusi/Highpass/HighpassH/Resonator84 ==
  In1 : Inport
  Constant : Constant  Value=0i
  Delay : Delay  DelayLength=1
  Gain : Gain  Gain=-0.99652+0.083308i
  GainH : Gain  Gain=-0.055575-0.99845i
  Real-Imag to Complex : RealImagToComplex
  Sum1 : Sum  Inputs=|++
  Out1 : Outport
  wires:
  Constant/1 -> Real-Imag to Complex/2
  Real-Imag to Complex/1 -> Sum1/1
  In1/1 -> Real-Imag to Complex/1
  GainH/1 -> Out1/1
  Gain/1 -> Sum1/2
  Delay/1 -> Gain/1
  Sum1/1 -> Delay/1, GainH/1

== system Filter_testaus_uusi/Highpass/HighpassH/Resonator85 ==
  In1 : Inport
  Constant : Constant  Value=0i
  Delay : Delay  DelayLength=1
  Gain : Gain  Gain=-0.99845+0.055575i
  GainH : Gain  Gain=0.04169+0.99913i
  Real-Imag to Complex : RealImagToComplex
  Sum1 : Sum  Inputs=|++
  Out1 : Outport
  wires:
  Constant/1 -> Real-Imag to Complex/2
  Real-Imag to Complex/1 -> Sum1/1
  In1/1 -> Real-Imag to Complex/1
  GainH/1 -> Out1/1
  Gain/1 -> Sum1/2
  Delay/1 -> Gain/1
  Sum1/1 -> Delay/1, GainH/1

== system Filter_testaus_uusi/Highpass/HighpassH/Resonator86 ==
  In1 : Inport
  Constant : Constant  Value=0i
  Delay : Delay  DelayLength=1
  Gain : Gain  Gain=-0.99961+0.027798i
  GainH : Gain  Gain=-0.027798-0.99961i
  Real-Imag to Complex : RealImagToComplex
  Sum1 : Sum  Inputs=|++
  Out1 : Outport
  wires:
  Constant/1 -> Real-Imag to Complex/2
  Real-Imag to Complex/1 -> Sum1/1
  In1/1 -> Real-Imag to Complex/1
  GainH/1 -> Out1/1
  Gain/1 -> Sum1/2
  Delay/1 -> Gain/1
  Sum1/1 -> Delay/1, GainH/1

== system Filter_testaus_uusi/Highpass/HighpassH/Resonator87 ==
  In1 : Inport
  Constant : Constant  Value=0i
  Delay : Delay  DelayLength=1
  Gain : Gain  Gain=-1+1.2246e-16i
  GainH : Gain  Gain=0.0139+0.9999i
  Real-Imag to Complex : RealImagToComplex
  Sum1 : Sum  Inputs=|++
  Out1 : Outport
  wires:
  Constant/1 -> Real-Imag to Complex/2
  Real-Imag to Complex/1 -> Sum1/1
  In1/1 -> Real-Imag to Complex/1
  GainH/1 -> Out1/1
  Gain/1 -> Sum1/2
  Delay/1 -> Gain/1
  Sum1/1 -> Delay/1, GainH/1

== system Filter_testaus_uusi/Highpass/HighpassH/Resonator88 ==
  In1 : Inport
  Constant : Constant  Value=0i
  Delay : Delay  DelayLength=1
  Gain : Gain  Gain=-0.99961-0.027798i
  GainH : Gain  Gain=1.9106e-14-1i
  Real-Imag to Complex : RealImagToComplex
  Sum1 : Sum  Inputs=|++
  Out1 : Outport
  wires:
  Constant/1 -> Real-Imag to Complex/2
  Real-Imag to Complex/1 -> Sum1/1
  In1/1 -> Real-Imag to Complex/1
  GainH/1 -> Out1/1
  Gain/1 -> Sum1/2
  Delay/1 -> Gain/1
  Sum1/1 -> Delay/1, GainH/1

== system Filter_testaus_uusi/Highpass/HighpassH/Resonator89 ==
  In1 : Inport
  Constant : Constant  Value=0i
  Delay : Delay  DelayLength=1
  Gain : Gain  Gain=-0.99845-0.055575i
  GainH : Gain  Gain=0.0139-0.9999i
  Real-Imag to Complex : RealImagToComplex
  Sum1 : Sum  Inputs=|++
  Out1 : Outport
  wires:
  Constant/1 -> Real-Imag to Complex/2
  Real-Imag to Complex/1 -> Sum1/1
  In1/1 -> Real-Imag to Complex/1
  GainH/1 -> Out1/1
  Gain/1 -> Sum1/2
  Delay/1 -> Gain/1
  Sum1/1 -> Delay/1, GainH/1

== system Filter_testaus_uusi/Highpass/HighpassH/Resonator9 ==
  In1 : Inport
  Constant : Constant  Value=0i
  Delay : Delay  DelayLength=1
  Gain : Gain  Gain=0.56277+0.82661i
  GainH : Gain  Gain=0.89037+0.45523i
  Real-Imag to Complex : RealImagToComplex
  Sum1 : Sum  Inputs=|++
  Out1 : Outport
  wires:
  Constant/1 -> Real-Imag to Complex/2
  Real-Imag to Complex/1 -> Sum1/1
  In1/1 -> Real-Imag to Complex/1
  GainH/1 -> Out1/1
  Gain/1 -> Sum1/2
  Delay/1 -> Gain/1
  Sum1/1 -> Delay/1, GainH/1

== system Filter_testaus_uusi/Highpass/HighpassH/Resonator90 ==
  In1 : Inport
  Constant : Constant  Value=0i
  Delay : Delay  DelayLength=1
  Gain : Gain  Gain=-0.99652-0.083308i
  GainH : Gain  Gain=-0.027798+0.99961i
  Real-Imag to Complex : RealImagToComplex
  Sum1 : Sum  Inputs=|++
  Out1 : Outport
  wires:
  Constant/1 -> Real-Imag to Complex/2
  Real-Imag to Complex/1 -> Sum1/1
  In1/1 -> Real-Imag to Complex/1
  GainH/1 -> Out1/1
  Gain/1 -> Sum1/2
  Delay/1 -> Gain/1
  Sum1/1 -> Delay/1, GainH/1

== system Filter_testaus_uusi/Highpass/HighpassH/Resonator91 ==
  In1 : Inport
  Constant : Constant  Value=0i
  Delay : Delay  DelayLength=1
  Gain : Gain  Gain=-0.99382-0.11098i
  GainH : Gain  Gain=0.04169-0.99913i
  Real-Imag to Complex : RealImagToComplex
  Sum1 : Sum  Inputs=|++
  Out1 : Outport
  wires:
  Constant/1 -> Real-Imag to Complex/2
  Real-Imag to Complex/1 -> Sum1/1
  In1/1 -> Real-Imag to Complex/1
  GainH/1 -> Out1/1
  Gain/1 -> Sum1/2
  Delay/1 -> Gain/1
  Sum1/1 -> Delay/1, GainH/1

== system Filter_testaus_uusi/Highpass/HighpassH/Resonator92 ==
  In1 : Inport
  Constant : Constant  Value=0i
  Delay : Delay  DelayLength=1
  Gain : Gain  Gain=-0.99035-0.13856i
  GainH : Gain  Gain=-0.055575+0.99845i
  Real-Imag to Complex : RealImagToComplex
  Sum1 : Sum  Inputs=|++
  Out1 : Outport
  wires:
  Constant/1 -> Real-Imag to Complex/2
  Real-Imag to Complex/1 -> Sum1/1
  In1/1 -> Real-Imag to Complex/1
  GainH/1 -> Out1/1
  Gain/1 -> Sum1/2
  Delay/1 -> Gain/1
  Sum1/1 -> Delay/1, GainH/1

== system Filter_testaus_uusi/Highpass/HighpassH/Resonator93 ==
  In1 : Inport
  Constant : Constant  Value=0i
  Delay : Delay  DelayLength=1
  Gain : Gain  Gain=-0.98612-0.16604i
  GainH : Gain  Gain=0.069448-0.99759i
  Real-Imag to Complex : RealImagToComplex
  Sum1 : Sum  Inputs=|++
  Out1 : Outport
  wires:
  Constant/1 -> Real-Imag to Complex/2
  Real-Imag to Complex/1 -> Sum1/1
  In1/1 -> Real-Imag to Complex/1
  GainH/1 -> Out1/1
  Gain/1 -> Sum1/2
  Delay/1 -> Gain/1
  Sum1/1 -> Delay/1, GainH/1

== system Filter_testaus_uusi/Highpass/HighpassH/Resonator94 ==
  In1 : Inport
  Constant : Constant  Value=0i
  Delay : Delay  DelayLength=1
  Gain : Gain  Gain=-0.98112-0.19339i
  GainH : Gain  Gain=-0.083308+0.99652i
  Real-Imag to Complex : RealImagToComplex
  Sum1 : Sum  Inputs=|++
  Out1 : Outport
  wires:
  Constant/1 -> Real-Imag to Complex/2
  Real-Imag to Complex/1 -> Sum1/1
  In1/1 -> Real-Imag to Complex/1
  GainH/1 -> Out1/1
  Gain/1 -> Sum1/2
  Delay/1 -> Gain/1
  Sum1/1 -> Delay/1, GainH/1

== system Filter_testaus_uusi/Highpass/HighpassH/Resonator95 ==
  In1 : Inport
  Constant : Constant  Value=0i
  Delay : Delay  DelayLength=1
  Gain : Gain  Gain=-0.97537-0.22058i
  GainH : Gain  Gain=0.097152-0.99527i
  Real-Imag to Complex : RealImagToComplex
  Sum1 : Sum  Inputs=|++
  Out1 : Outport
  wires:
  Constant/1 -> Real-Imag to Complex/2
  Real-Imag to Complex/1 -> Sum1/1
  In1/1 -> Real-Imag to Complex/1
  GainH/1 -> Out1/1
  Gain/1 -> Sum1/2
  Delay/1 -> Gain/1
  Sum1/1 -> Delay/1, GainH/1

== system Filter_testaus_uusi/Highpass/HighpassH/Resonator96 ==
  In1 : Inport
  Constant : Constant  Value=0i
  Delay : Delay  DelayLength=1
  Gain : Gain  Gain=-0.96886-0.24761i
  GainH : Gain  Gain=-0.11098+0.99382i
  Real-Imag to Complex : RealImagToComplex
  Sum1 : Sum  Inputs=|++
  Out1 : Outport
  wires:
  Constant/1 -> Real-Imag to Complex/2
  Real-Imag to Complex/1 -> Sum1/1
  In1/1 -> Real-Imag to Complex/1
  GainH/1 -> Out1/1
  Gain/1 -> Sum1/2
  Delay/1 -> Gain/1
  Sum1/1 -> Delay/1, GainH/1

== system Filter_testaus_uusi/Highpass/HighpassH/Resonator97 ==
  In1 : Inport
  Constant : Constant  Value=0i
  Delay : Delay  DelayLength=1
  Gain : Gain  Gain=-0.9616-0.27445i
  GainH : Gain  Gain=0.12478-0.99218i
  Real-Imag to Complex : RealImagToComplex
  Sum1 : Sum  Inputs=|++
  Out1 : Outport
  wires:
  Constant/1 -> Real-Imag to Complex/2
  Real-Imag to Complex/1 -> Sum1/1
  In1/1 -> Real-Imag to Complex/1
  GainH/1 -> Out1/1
  Gain/1 -> Sum1/2
  Delay/1 -> Gain/1
  Sum1/1 -> Delay/1, GainH/1

== system Filter_testaus_uusi/Highpass/HighpassH/Resonator98 ==
  In1 : Inport
  Constant : Constant  Value=0i
  Delay : Delay  DelayLength=1
  Gain : Gain  Gain=-0.9536-0.30107i
  GainH : Gain  Gain=-0.13856+0.99035i
  Real-Imag to Complex : RealImagToComplex
  Sum1 : Sum  Inputs=|++
  Out1 : Outport
  wires:
  Constant/1 -> Real-Imag to Complex/2
  Real-Imag to Complex/1 -> Sum1/1
  In1/1 -> Real-Imag to Complex/1
  GainH/1 -> Out1/1
  Gain/1 -> Sum1/2
  Delay/1 -> Gain/1
  Sum1/1 -> Delay/1, GainH/1

== system Filter_testaus_uusi/Highpass/HighpassH/Resonator99 ==
  In1 : Inport
  Constant : Constant  Value=0i
  Delay : Delay  DelayLength=1
  Gain : Gain  Gain=-0.94486-0.32747i
  GainH : Gain  Gain=0.15231-0.98833i
  Real-Imag to Complex : RealImagToComplex
  Sum1 : Sum  Inputs=|++
  Out1 : Outport
  wires:
  Constant/1 -> Real-Imag to Complex/2
  Real-Imag to Complex/1 -> Sum1/1
  In1/1 -> Real-Imag to Complex/1
  GainH/1 -> Out1/1
  Gain/1 -> Sum1/2
  Delay/1 -> Gain/1
  Sum1/1 -> Delay/1, GainH/1

== system Filter_testaus_uusi/Highpass/HighpassH/ResonatorTemplate ==
  In1 : Inport
  Constant : Constant  Value=0i
  Delay : Delay  DelayLength=1
  Gain : Gain
  GainH : Gain
  Real-Imag to Complex : RealImagToComplex
  Sum1 : Sum  Inputs=|++
  Out1 : Outport
  wires:
  Sum1/1 -> GainH/1, Delay/1
  Delay/1 -> Gain/1
  Gain/1 -> Sum1/2
  GainH/1 -> Out1/1
  In1/1 -> Real-Imag to Complex/1
  Real-Imag to Complex/1 -> Sum1/1
  Constant/1 -> Real-Imag to Complex/2

== system Filter_testaus_uusi/Lowpass/LowpassH/Resonator1 ==
  In1 : Inport
  Constant : Constant  Value=0i
  Delay : Delay  DelayLength=1
  Gain : Gain  Gain=0.99961+0.027798i
  GainH : Gain
  Real-Imag to Complex : RealImagToComplex
  Sum1 : Sum  Inputs=|++
  Out1 : Outport
  wires:
  Constant/1 -> Real-Imag to Complex/2
  In1/1 -> Real-Imag to Complex/1
  Real-Imag to Complex/1 -> Sum1/1
  GainH/1 -> Out1/1
  Gain/1 -> Sum1/2
  Delay/1 -> Gain/1
  Sum1/1 -> Delay/1, GainH/1

== system Filter_testaus_uusi/Lowpass/LowpassH/Resonator10 ==
  In1 : Inport
  Constant : Constant  Value=0i
  Delay : Delay  DelayLength=1
  Gain : Gain  Gain=0.9616+0.27445i
  GainH : Gain  Gain=0.72887-0.68465i
  Real-Imag to Complex : RealImagToComplex
  Sum1 : Sum  Inputs=|++
  Out1 : Outport
  wires:
  Constant/1 -> Real-Imag to Complex/2
  In1/1 -> Real-Imag to Complex/1
  Real-Imag to Complex/1 -> Sum1/1
  GainH/1 -> Out1/1
  Gain/1 -> Sum1/2
  Delay/1 -> Gain/1
  Sum1/1 -> Delay/1, GainH/1

== system Filter_testaus_uusi/Lowpass/LowpassH/Resonator11 ==
  In1 : Inport
  Constant : Constant  Value=0i
  Delay : Delay  DelayLength=1
  Gain : Gain  Gain=0.9536+0.30107i
  GainH : Gain  Gain=0.034745-0.9994i
  Real-Imag to Complex : RealImagToComplex
  Sum1 : Sum  Inputs=|++
  Out1 : Outport
  wires:
  Constant/1 -> Real-Imag to Complex/2
  In1/1 -> Real-Imag to Complex/1
  Real-Imag to Complex/1 -> Sum1/1
  GainH/1 -> Out1/1
  Gain/1 -> Sum1/2
  Delay/1 -> Gain/1
  Sum1/1 -> Delay/1, GainH/1

== system Filter_testaus_uusi/Lowpass/LowpassH/Resonator12 ==
  In1 : Inport
  Constant : Constant  Value=0i
  Delay : Delay  DelayLength=1
  Gain : Gain  Gain=0.94486+0.32747i
  GainH : Gain  Gain=-0.67957-0.73361i
  Real-Imag to Complex : RealImagToComplex
  Sum1 : Sum  Inputs=|++
  Out1 : Outport
  wires:
  Constant/1 -> Real-Imag to Complex/2
  In1/1 -> Real-Imag to Complex/1
  Real-Imag to Complex/1 -> Sum1/1
  GainH/1 -> Out1/1
  Gain/1 -> Sum1/2
  Delay/1 -> Gain/1
  Sum1/1 -> Delay/1, GainH/1

== system Filter_testaus_uusi/Lowpass/LowpassH/Resonator13 ==
  In1 : Inport
  Constant : Constant  Value=0i
  Delay : Delay  DelayLength=1
  Gain : Gain  Gain=0.9616-0.27445i
  GainH : Gain  Gain=-0.67957+0.73361i
  Real-Imag to Complex : RealImagToComplex
  Sum1 : Sum  Inputs=|++
  Out1 : Outport
  wires:
  Constant/1 -> Real-Imag to Complex/2
  In1/1 -> Real-Imag to Complex/1
  Real-Imag to Complex/1 -> Sum1/1
  GainH/1 -> Out1/1
  Gain/1 -> Sum1/2
  Delay/1 -> Gain/1
  Sum1/1 -> Delay/1, GainH/1

== system Filter_testaus_uusi/Lowpass/LowpassH/Resonator14 ==
  In1 : Inport
  Constant : Constant  Value=0i
  Delay : Delay  DelayLength=1
  Gain : Gain  Gain=0.96886-0.24761i
  GainH : Gain  Gain=0.034745+0.9994i
  Real-Imag to Complex : RealImagToComplex
  Sum1 : Sum  Inputs=|++
  Out1 : Outport
  wires:
  Constant/1 -> Real-Imag to Complex/2
  In1/1 -> Real-Imag to Complex/1
  Real-Imag to Complex/1 -> Sum1/1
  GainH/1 -> Out1/1
  Gain/1 -> Sum1/2
  Delay/1 -> Gain/1
  Sum1/1 -> Delay/1, GainH/1

== system Filter_testaus_uusi/Lowpass/LowpassH/Resonator15 ==
  In1 : Inport
  Constant : Constant  Value=0i
  Delay : Delay  DelayLength=1
  Gain : Gain  Gain=0.97537-0.22058i
  GainH : Gain  Gain=0.72887+0.68465i
  Real-Imag to Complex : RealImagToComplex
  Sum1 : Sum  Inputs=|++
  Out1 : Outport
  wires:
  Constant/1 -> Real-Imag to Complex/2
  In1/1 -> Real-Imag to Complex/1
  Real-Imag to Complex/1 -> Sum1/1
  GainH/1 -> Out1/1
  Gain/1 -> Sum1/2
  Delay/1 -> Gain/1
  Sum1/1 -> Delay/1, GainH/1

== system Filter_testaus_uusi/Lowpass/LowpassH/Resonator16 ==
  In1 : Inport
  Constant : Constant  Value=0i
  Delay : Delay  DelayLength=1
  Gain : Gain  Gain=0.98112-0.19339i
  GainH : Gain  Gain=0.99961-0.027798i
  Real-Imag to Complex : RealImagToComplex
  Sum1 : Sum  Inputs=|++
  Out1 : Outport
  wires:
  Constant/1 -> Real-Imag to Complex/2
  In1/1 -> Real-Imag to Complex/1
  Real-Imag to Complex/1 -> Sum1/1
  GainH/1 -> Out1/1
  Gain/1 -> Sum1/2
  Delay/1 -> Gain/1
  Sum1/1 -> Delay/1, GainH/1

== system Filter_testaus_uusi/Lowpass/LowpassH/Resonator17 ==
  In1 : Inport
  Constant : Constant  Value=0i
  Delay : Delay  DelayLength=1
  Gain : Gain  Gain=0.98612-0.16604i
  GainH : Gain  Gain=0.6897-0.7241i
  Real-Imag to Complex : RealImagToComplex
  Sum1 : Sum  Inputs=|++
  Out1 : Outport
  wires:
  Constant/1 -> Real-Imag to Complex/2
  In1/1 -> Real-Imag to Complex/1
  Real-Imag to Complex/1 -> Sum1/1
  GainH/1 -> Out1/1
  Gain/1 -> Sum1/2
  Delay/1 -> Gain/1
  Sum1/1 -> Delay/1, GainH/1

== system Filter_testaus_uusi/Lowpass/LowpassH/Resonator18 ==
  In1 : Inport
  Constant : Constant  Value=0i
  Delay : Delay  DelayLength=1
  Gain : Gain  Gain=0.99035-0.13856i
  GainH : Gain  Gain=-0.02085-0.99978i
  Real-Imag to Complex : RealImagToComplex
  Sum1 : Sum  Inputs=|++
  Out1 : Outport
  wires:
  Constant/1 -> Real-Imag to Complex/2
  In1/1 -> Real-Imag to Complex/1
  Real-Imag to Complex/1 -> Sum1/1
  GainH/1 -> Out1/1
  Gain/1 -> Sum1/2
  Delay/1 -> Gain/1
  Sum1/1 -> Delay/1, GainH/1

== system Filter_testaus_uusi/Lowpass/LowpassH/Resonator19 ==
  In1 : Inport
  Constant : Constant  Value=0i
  Delay : Delay  DelayLength=1
  Gain : Gain  Gain=0.99382-0.11098i
  GainH : Gain  Gain=-0.71929-0.69471i
  Real-Imag to Complex : RealImagToComplex
  Sum1 : Sum  Inputs=|++
  Out1 : Outport
  wires:
  Constant/1 -> Real-Imag to Complex/2
  In1/1 -> Real-Imag to Complex/1
  Real-Imag to Complex/1 -> Sum1/1
  GainH/1 -> Out1/1
  Gain/1 -> Sum1/2
  Delay/1 -> Gain/1
  Sum1/1 -> Delay/1, GainH/1

== system Filter_testaus_uusi/Lowpass/LowpassH/Resonator2 ==
  In1 : Inport
  Constant : Constant  Value=0i
  Delay : Delay  DelayLength=1
  Gain : Gain  Gain=0.99845+0.055575i
  GainH : Gain  Gain=0.70956-0.70465i
  Real-Imag to Complex : RealImagToComplex
  Sum1 : Sum  Inputs=|++
  Out1 : Outport
  wires:
  Constant/1 -> Real-Imag to Complex/2
  In1/1 -> Real-Imag to Complex/1
  Real-Imag to Complex/1 -> Sum1/1
  GainH/1 -> Out1/1
  Gain/1 -> Sum1/2
  Delay/1 -> Gain/1
  Sum1/1 -> Delay/1, GainH/1

== system Filter_testaus_uusi/Lowpass/LowpassH/Resonator20 ==
  In1 : Inport
  Constant : Constant  Value=0i
  Delay : Delay  DelayLength=1
  Gain : Gain  Gain=0.99652-0.083308i
  GainH : Gain  Gain=-0.9999+0.0139i
  Real-Imag to Complex : RealImagToComplex
  Sum1 : Sum  Inputs=|++
  Out1 : Outport
  wires:
  Constant/1 -> Real-Imag to Complex/2
  In1/1 -> Real-Imag to Complex/1
  Real-Imag to Complex/1 -> Sum1/1
  GainH/1 -> Out1/1
  Gain/1 -> Sum1/2
  Delay/1 -> Gain/1
  Sum1/1 -> Delay/1, GainH/1

== system Filter_testaus_uusi/Lowpass/LowpassH/Resonator21 ==
  In1 : Inport
  Constant : Constant  Value=0i
  Delay : Delay  DelayLength=1
  Gain : Gain  Gain=0.99845-0.055575i
  GainH : Gain  Gain=-0.6997+0.71444i
  Real-Imag to Complex : RealImagToComplex
  Sum1 : Sum  Inputs=|++
  Out1 : Outport
  wires:
  Constant/1 -> Real-Imag to Complex/2
  In1/1 -> Real-Imag to Complex/1
  Real-Imag to Complex/1 -> Sum1/1
  GainH/1 -> Out1/1
  Gain/1 -> Sum1/2
  Delay/1 -> Gain/1
  Sum1/1 -> Delay/1, GainH/1

== system Filter_testaus_uusi/Lowpass/LowpassH/Resonator22 ==
  In1 : Inport
  Constant : Constant  Value=0i
  Delay : Delay  DelayLength=1
  Gain : Gain  Gain=0.99961-0.027798i
  GainH : Gain  Gain=0.0069504+0.99998i
  Real-Imag to Complex : RealImagToComplex
  Sum1 : Sum  Inputs=|++
  Out1 : Outport
  wires:
  Constant/1 -> Real-Imag to Complex/2
  In1/1 -> Real-Imag to Complex/1
  Real-Imag to Complex/1 -> Sum1/1
  GainH/1 -> Out1/1
  Gain/1 -> Sum1/2
  Delay/1 -> Gain/1
  Sum1/1 -> Delay/1, GainH/1

== system Filter_testaus_uusi/Lowpass/LowpassH/Resonator23 ==
  In1 : Inport
  Constant : Constant  Value=0i
  Delay : Delay  DelayLength=1
  Gain : Gain  Gain=1-2.4493e-16i
  GainH : Gain  Gain=0.70956+0.70465i
  Real-Imag to Complex : RealImagToComplex
  Sum1 : Sum  Inputs=|++
  Out1 : Outport
  wires:
  Constant/1 -> Real-Imag to Complex/2
  In1/1 -> Real-Imag to Complex/1
  Real-Imag to Complex/1 -> Sum1/1
  GainH/1 -> Out1/1
  Gain/1 -> Sum1/2
  Delay/1 -> Gain/1
  Sum1/1 -> Delay/1, GainH/1

== system Filter_testaus_uusi/Lowpass/LowpassH/Resonator3 ==
  In1 : Inport
  Constant : Constant  Value=0i
  Delay : Delay  DelayLength=1
  Gain : Gain  Gain=0.99652+0.083308i
  GainH : Gain  Gain=0.0069504-0.99998i
  Real-Imag to Complex : RealImagToComplex
  Sum1 : Sum  Inputs=|++
  Out1 : Outport
  wires:
  Constant/1 -> Real-Imag to Complex/2
  In1/1 -> Real-Imag to Complex/1
  Real-Imag to Complex/1 -> Sum1/1
  GainH/1 -> Out1/1
  Gain/1 -> Sum1/2
  Delay/1 -> Gain/1
  Sum1/1 -> Delay/1, GainH/1

== system Filter_testaus_uusi/Lowpass/LowpassH/Resonator4 ==
  In1 : Inport
  Constant : Constant  Value=0i
  Delay : Delay  DelayLength=1
  Gain : Gain  Gain=0.99382+0.11098i
  GainH : Gain  Gain=-0.6997-0.71444i
  Real-Imag to Complex : RealImagToComplex
  Sum1 : Sum  Inputs=|++
  Out1 : Outport
  wires:
  Constant/1 -> Real-Imag to Complex/2
  In1/1 -> Real-Imag to Complex/1
  Real-Imag to Complex/1 -> Sum1/1
  GainH/1 -> Out1/1
  Gain/1 -> Sum1/2
  Delay/1 -> Gain/1
  Sum1/1 -> Delay/1, GainH/1

== system Filter_testaus_uusi/Lowpass/LowpassH/Resonator5 ==
  In1 : Inport
  Constant : Constant  Value=0i
  Delay : Delay  DelayLength=1
  Gain : Gain  Gain=0.99035+0.13856i
  GainH : Gain  Gain=-0.9999-0.0139i
  Real-Imag to Complex : RealImagToComplex
  Sum1 : Sum  Inputs=|++
  Out1 : Outport
  wires:
  Constant/1 -> Real-Imag to Complex/2
  In1/1 -> Real-Imag to Complex/1
  Real-Imag to Complex/1 -> Sum1/1
  GainH/1 -> Out1/1
  Gain/1 -> Sum1/2
  Delay/1 -> Gain/1
  Sum1/1 -> Delay/1, GainH/1

== system Filter_testaus_uusi/Lowpass/LowpassH/Resonator6 ==
  In1 : Inport
  Constant : Constant  Value=0i
  Delay : Delay  DelayLength=1
  Gain : Gain  Gain=0.98612+0.16604i
  GainH : Gain  Gain=-0.71929+0.69471i
  Real-Imag to Complex : RealImagToComplex
  Sum1 : Sum  Inputs=|++
  Out1 : Outport
  wires:
  Constant/1 -> Real-Imag to Complex/2
  In1/1 -> Real-Imag to Complex/1
  Real-Imag to Complex/1 -> Sum1/1
  GainH/1 -> Out1/1
  Gain/1 -> Sum1/2
  Delay/1 -> Gain/1
  Sum1/1 -> Delay/1, GainH/1

== system Filter_testaus_uusi/Lowpass/LowpassH/Resonator7 ==
  In1 : Inport
  Constant : Constant  Value=0i
  Delay : Delay  DelayLength=1
  Gain : Gain  Gain=0.98112+0.19339i
  GainH : Gain  Gain=-0.02085+0.99978i
  Real-Imag to Complex : RealImagToComplex
  Sum1 : Sum  Inputs=|++
  Out1 : Outport
  wires:
  Constant/1 -> Real-Imag to Complex/2
  In1/1 -> Real-Imag to Complex/1
  Real-Imag to Complex/1 -> Sum1/1
  GainH/1 -> Out1/1
  Gain/1 -> Sum1/2
  Delay/1 -> Gain/1
  Sum1/1 -> Delay/1, GainH/1
